simulink model "cpu_ctlr"  (Simulink 7.1)
settings: Solver=FixedStepDiscrete  StartTime=0.0  StopTime=200  FixedStep=1  RelTol=1e-3
libraries: simulink x1
settings Model: Creator=vak  LastModifiedBy=vak
settings DebuggingCC: AlgebraicLoopMsg=none  ArtificialAlgebraicLoopMsg=none  SolverPrmCheckMsg=error  DiscreteInheritContinuousMsg=error

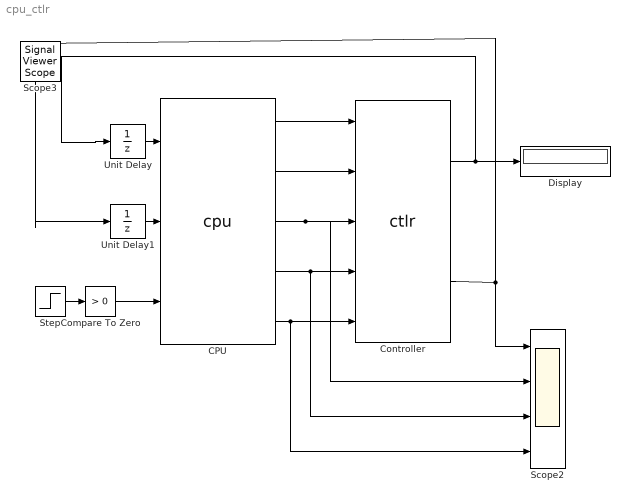
== system cpu_ctlr ==
  CPU : S-Function  FunctionName=cpu  SFunctionModules='cpu-sfun node1'  EnableBusSupport=off
      mask Display: port_label('input',1,'datain')port_label('input',2,'ack')port_label('input',3,'rst')port_label('output',1,'dataout')port_label('output',2,'addr')port_label('output',3,'rd')port_label('output',4,'wrh')port_label('output',5,'wrl')
  Compare To Zero : simulink/Logic and Bit Operations/Compare To Zero  SystemSampleTime=-1  relop=>  LogicOutDataTypeMode=boolean  ZeroCross=off
  Controller : S-Function  FunctionName=ctlr  SFunctionModules='ctlr-sfun ctlr'  EnableBusSupport=off
      mask Display: port_label('input',1,'datain')port_label('input',2,'addr')port_label('input',3,'rd')port_label('input',4,'wrh')port_label('input',5,'wrl')port_label('output',1,'dataout')port_label('output',2,'ack')
  Display : Display
      settings: Format=hex (Stored Integer)
  Scope2 : Scope  NumInputPorts=4
      settings: YMin=-5~-5~-5~-5  YMax=5~5~5~5  SaveName=ScopeData2
  Step : Step  Before=1  After=0  SampleTime=0  VectorParams1D=off
  Unit Delay : UnitDelay
  Unit Delay1 : UnitDelay
  Scope3 : SignalViewerScope  IOType=viewer  RefreshTime=0.035000
  wires:
  Step/1 -> Compare To Zero/1
  Compare To Zero/1 -> CPU/3
  CPU/1 -> Controller/1
  CPU/2 -> Controller/2
  CPU/3 -> Controller/3, Scope2/2
  CPU/4 -> Controller/4, Scope2/3
  CPU/5 -> Controller/5, Scope2/4
  Controller/1 -> Display/1, Unit Delay/1
  Controller/2 -> Unit Delay1/1, Scope2/1
  Unit Delay/1 -> CPU/1
  Unit Delay1/1 -> CPU/2
